simulink model "intersection_continous"  (R2021a)
settings: Solver=VariableStepAuto  StartTime=0.0  StopTime=10.0  RelTol=1e-3
values from neighbouring files (symbols this model uses):
  Ax = [X_RobotT(:);X_Robot1T(:);X_Robot2T(:)]    [path_obst.m]
  Ay = [Y_RobotT(:);Y_Robot1T(:);Y_Robot2T(:)]    [path_obst.m]
  Ox = obst(:,1)    [path_obst.m]
  Oy = obst(:,2)    [path_obst.m]

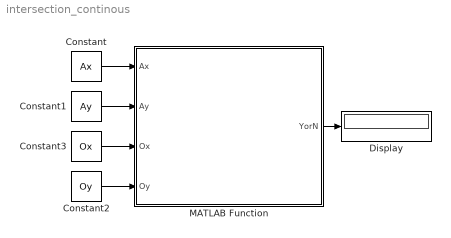
== system intersection_continous ==
  Constant : Constant  Value=Ax
  Constant1 : Constant  Value=Ay
  Constant2 : Constant  Value=Oy
  Constant3 : Constant  Value=Ox
  Display : Display
  MATLAB Function : MATLAB Function  TreatAsAtomicUnit=on
  wires:
  Constant/1 -> MATLAB Function/1(Ax)
  Constant1/1 -> MATLAB Function/2(Ay)
  Constant2/1 -> MATLAB Function/4(Oy)
  Constant3/1 -> MATLAB Function/3(Ox)
  MATLAB Function/1(YorN) -> Display/1

== matlab function intersection_continous/MATLAB Function ==
function YorN = fcn(Ax,Ay,Ox,Oy)
s1=size(Ax);
s2=size(Ox);
a1=zeros(s1(1),1);
b1=zeros(s1(1),1);
c1=zeros(s1(1),1);
a2=zeros(s2(1),1);
b2=zeros(s2(1),1);
c2=zeros(s2(1),1);
YorN=0;
for n=1:s1(1)
   if n < s1(1)
     post_n=n+1;
   else
     post_n=1; 
   end
   a1(n) = Ay(post_n) - Ay(n);
   b1(n) = Ax(n) - Ax(post_n);
   c1(n) = a1(n)*Ax(n) + b1(n)*Ay(n);
end    
for i=1:s2(1)
   if i < s2(1)
    post_i=i+1;
   else
    post_i=1; 
   end
   a2(i) = Oy(post_i) - Oy(i);
   b2(i) = Ox(i) - Ox(post_i);
   c2(i) = a2(i)*Ox(i) + b2(i)*Oy(i);
 end    
for i=1:s2(1)
    for n=1:s1(1)
     if i < s2(1)
       post_i=i+1;
     else
       post_i=1; 
     end
     
     if n < s1(1)
       post_n=n+1;
     else
       post_n=1; 
     end
     
     if (a1(n)*b2(i) - a2(i)*b1(n))==0
       X =inf;    
     else
       X =(b2(i)*c1(n) - b1(n)*c2(i))/(a1(n)*b2(i) - a2(i)*b1(n));
     end
     if X > max(Ax(n),Ax(post_n))|| X < min(Ax(n),Ax(post_n))|| X > max(Ox(i),Ox(post_i))|| X < min(Ox(i),Ox(post_i))
     else
          YorN=1;
     end
   end
end
